simulink model "simple_RC_Circuit"  (R2021a)
settings: Solver=VariableStepAuto  StartTime=0.0  StopTime=10.0  MaxStep=1e-3  RelTol=1e-3
values from neighbouring files (symbols this model uses):
  C = 1e-6    (= 1e-06)    [simple_RC_Circuit_int.m]
  R = 50    [simple_RC_Circuit_int.m]
settings Model: Creator=lenovo  LastModifiedBy=lenovo

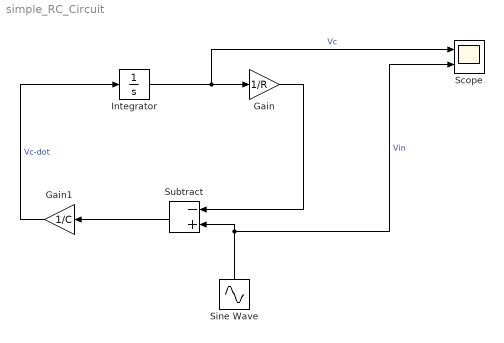
== system simple_RC_Circuit ==
  Gain : Gain  Gain=1/R
  Gain1 : Gain  Gain=1/C
  Integrator : Integrator  InitialCondition=3
  Scope : Scope  NumInputPorts=2
  Sine Wave : Sin  Amplitude=5  Frequency=2*pi  SampleTime=0
  Subtract : Sum  Inputs=-+
  wires:
  Gain1/1 -> Integrator/1  "Vc-dot"
  Integrator/1 -> Scope/1, Gain/1  "Vc"
  Subtract/1 -> Gain1/1
  Sine Wave/1 -> Subtract/2, Scope/2  "Vin"
  Gain/1 -> Subtract/1
